simulink model "Simulation_Laboratory_Crazyflie2_X"  (R2015b)
settings: Solver=FixedStepAuto  SolverMode=SingleTasking  StartTime=0.0  StopTime=50  FixedStep=0.01  RelTol=1e-3
values from neighbouring files (symbols this model uses):
  fm = 0.2685    [CRAZYFLIE_SETUP.m]
  fs_inner = 50    [CRAZYFLIE_SETUP.m]
  fs_outer = 25    [CRAZYFLIE_SETUP.m]
  g = 9.81    [CRAZYFLIE_SETUP.m]
  Ixx = 1.657e-5    (= 1.657e-05)    [CRAZYFLIE_SETUP.m]
  Iyy = 1.665e-5    (= 1.665e-05)    [CRAZYFLIE_SETUP.m]
  Izz = 2.296e-5    (= 2.296e-05)    [CRAZYFLIE_SETUP.m]
  KDp = 2.5    [CRAZYFLIE_SETUP.m]
  KDphi = 0.3    [CRAZYFLIE_SETUP.m]
  KDq = 2.5    [CRAZYFLIE_SETUP.m]
  KDr = 2.5    [CRAZYFLIE_SETUP.m]
  KDtheta = 0.3    [CRAZYFLIE_SETUP.m]
  KIp = 500    [CRAZYFLIE_SETUP.m]
  KIphi = 0.3    [CRAZYFLIE_SETUP.m]
  KIq = 500    [CRAZYFLIE_SETUP.m]
  KIr = 500    [CRAZYFLIE_SETUP.m]
  KItheta = 0.3    [CRAZYFLIE_SETUP.m]
  KPp = 250    [CRAZYFLIE_SETUP.m]
  KPphi = 1.0    (= 1)    [CRAZYFLIE_SETUP.m]
  KPq = 250    [CRAZYFLIE_SETUP.m]
  KPr = 250    [CRAZYFLIE_SETUP.m]
  KPtheta = 1.0    (= 1)    [CRAZYFLIE_SETUP.m]
  m = 0.027    [CRAZYFLIE_SETUP.m]
  MCO1 = [1,-1/2,-1/2,-1 ... (first row only)    [CRAZYFLIE_SETUP.m]
  ML1 = 2*we*[CT,CT,CT,CT ... (first row only)    [CRAZYFLIE_SETUP.m]
  ML2 = [0,0 ... (first row only)    [CRAZYFLIE_SETUP.m]
  ML3 = [1/m;0]    [CRAZYFLIE_SETUP.m]
  ML4 = [0,0 ... (first row only)    [CRAZYFLIE_SETUP.m]
  ML5 = [1/Izz;0]    [CRAZYFLIE_SETUP.m]
  ML6 = [0,0,0,0 ... (first row only)    [CRAZYFLIE_SETUP.m]
  ML7 = [1/Ixx;0;0;0]    [CRAZYFLIE_SETUP.m]
  ML8 = [0,0,0,0 ... (first row only)    [CRAZYFLIE_SETUP.m]
  ML9 = [1/Iyy;0;0;0]    [CRAZYFLIE_SETUP.m]
  MNL1 = [CT,CT,CT,CT ... (first row only)    [CRAZYFLIE_SETUP.m]
  PWMe = (we-4070.3)/0.2685    [CRAZYFLIE_SETUP.m]
libraries: simulink x2
settings Model: Creator=Rafael  LastModifiedBy=Rafael
settings DataIOCC: SaveFormat=Array  SignalLoggingSaveFormat=ModelDataLogs
settings OptimizationCC: ExpressionDepthLimit=2147483647
settings DebuggingCC: UnderspecifiedInitializationDetection=Classic  MergeDetectMultiDrivingBlocksExec=none  SolverPrmCheckMsg=warning  FcnCallInpInsideContextMsg=EnableAllAsWarning  StateNameClashWarn=warning
settings HardwareCC: ProdBitPerPointer=32  ProdLargestAtomicFloat=None  ProdIntDivRoundTo=Undefined  ProdEndianess=Unspecified  ProdWordSize=32  ProdHWDeviceType=32-bit Generic
settings GRTTargetCC: GeneratePreprocessorConditionals=Disable all
settings ConfigComp: CovModelRefEnable=Off

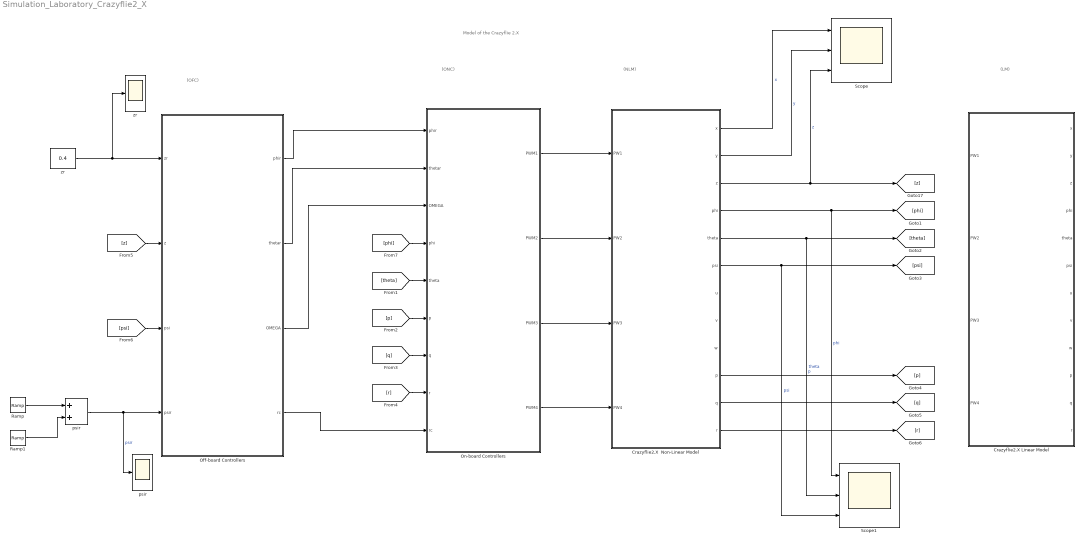
== system Simulation_Laboratory_Crazyflie2_X ==
  note: (NLM)
  note: Model of the Crazyflie 2.X
  note: (ONC)
  note: (LM)
  note: (OFC)
  " zr" : Scope
  Crazyflie2.X  Non-Linear Model : Subsystem
  Crazyflie2.X Linear Model : Subsystem
  Off-board Controllers : Subsystem
  On-board Controllers : Subsystem
  Ramp : simulink/Sources/Ramp  slope=15  start=5  X0=0
  Ramp1 : simulink/Sources/Ramp  slope=-15  start=11  X0=0
  Scope : Scope  NumInputPorts=3
  Scope1 : Scope  NumInputPorts=3
  psir : Sum
  "psir " : Scope
  zr : Constant  Value=0.4
  wires:
  [phi] -> On-board Controllers/4(phi)
  [theta] -> On-board Controllers/5(theta)
  [p] -> On-board Controllers/6(p)
  [q] -> On-board Controllers/7(q)
  [r] -> On-board Controllers/8(r)
  [z] -> Off-board Controllers/2(z)
  [psi] -> Off-board Controllers/3(psi)
  Crazyflie2.X  Non-Linear Model/11(q) -> [q]
  Crazyflie2.X  Non-Linear Model/3(z) -> [z], Scope/3  "z"
  Crazyflie2.X  Non-Linear Model/12(r) -> [r]
  zr/1 -> " zr"/1, Off-board Controllers/1(zr)
  Off-board Controllers/1(phir) -> On-board Controllers/1(phir)
  Crazyflie2.X  Non-Linear Model/10(p) -> [p]  "p"
  On-board Controllers/1(PWM1) -> Crazyflie2.X  Non-Linear Model/1(PW1)
  On-board Controllers/2(PWM2) -> Crazyflie2.X  Non-Linear Model/2(PW2)
  On-board Controllers/4(PWM4) -> Crazyflie2.X  Non-Linear Model/4(PW4)
  On-board Controllers/3(PWM3) -> Crazyflie2.X  Non-Linear Model/3(PW3)
  Crazyflie2.X  Non-Linear Model/4(phi) -> Scope1/1, [phi]  "phi"
  Crazyflie2.X  Non-Linear Model/5(theta) -> [theta], Scope1/2  "theta"
  Crazyflie2.X  Non-Linear Model/6(psi) -> [psi], Scope1/3  "psi"
  Off-board Controllers/2(thetar) -> On-board Controllers/2(thetar)
  Off-board Controllers/3(OMEGA) -> On-board Controllers/3(OMEGA)
  Off-board Controllers/4(rc) -> On-board Controllers/9(rc)
  Ramp/1 -> psir/1
  Ramp1/1 -> psir/2
  psir/1 -> "psir "/1, Off-board Controllers/4(psir)  "psir"
  Crazyflie2.X  Non-Linear Model/1(x) -> Scope/1  "x"
  Crazyflie2.X  Non-Linear Model/2(y) -> Scope/2  "y"

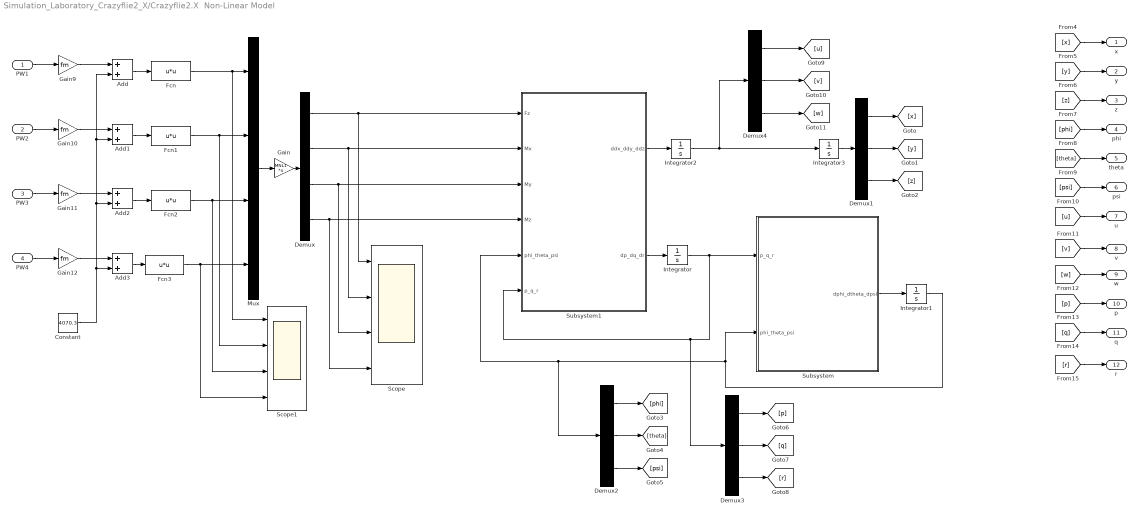
== system Simulation_Laboratory_Crazyflie2_X/Crazyflie2.X  Non-Linear Model ==
  PW1 : Inport
  PW2 : Inport  Port=2
  PW3 : Inport  Port=3
  PW4 : Inport  Port=4
  Add{,1..3} (4 alike) : Sum
  Constant : Constant  Value=4070.3
  Demux : Demux
  Demux{1..4} (4 alike) : Demux  Outputs=3
  Fcn{,1..3} (4 alike) : Fcn  Expr=u*u
  Gain : Gain  Gain=MNL1  Multiplication=Matrix(K*u) (u vector)
  Gain{9..12} (4 alike) : Gain  Gain=fm
  Integrator{,1..3} (4 alike) : Integrator
  Mux : Mux
  Scope : Scope  NumInputPorts=4
  Scope1 : Scope  NumInputPorts=4
  Subsystem : Subsystem
  Subsystem1 : Subsystem
  x : Outport
  y : Outport  Port=2
  z : Outport  Port=3
  phi : Outport  Port=4
  theta : Outport  Port=5
  psi : Outport  Port=6
  u : Outport  Port=7
  v : Outport  Port=8
  w : Outport  Port=9
  p : Outport  Port=10
  q : Outport  Port=11
  r : Outport  Port=12
  wires:
  Mux/1 -> Gain/1
  Gain/1 -> Demux/1
  Demux/1 -> Scope/1, Subsystem1/1(Fz)
  Demux/2 -> Scope/2, Subsystem1/2(Mx)
  Demux/3 -> Scope/3, Subsystem1/3(My)
  Demux/4 -> Scope/4, Subsystem1/4(Mz)
  [x] -> x/1
  [y] -> y/1
  [z] -> z/1
  [phi] -> phi/1
  [theta] -> theta/1
  [psi] -> psi/1
  [u] -> u/1
  [v] -> v/1
  [w] -> w/1
  [p] -> p/1
  [q] -> q/1
  [r] -> r/1
  PW1/1 -> Gain9/1
  PW2/1 -> Gain10/1
  PW3/1 -> Gain11/1
  PW4/1 -> Gain12/1
  Subsystem1/2(dp_dq_dr) -> Integrator/1
  Integrator/1 -> Subsystem/1(p_q_r), Subsystem1/6(p_q_r), Demux3/1
  Subsystem/1(dphi_dtheta_dpsi) -> Integrator1/1
  Integrator1/1 -> Subsystem/2(phi_theta_psi), Subsystem1/5(phi_theta_psi), Demux2/1
  Subsystem1/1(ddx_ddy_ddz) -> Integrator2/1
  Integrator2/1 -> Integrator3/1, Demux4/1
  Integrator3/1 -> Demux1/1
  Demux1/1 -> [x]
  Demux1/2 -> [y]
  Demux1/3 -> [z]
  Fcn/1 -> Mux/1, Scope1/1
  Fcn1/1 -> Mux/2, Scope1/2
  Fcn2/1 -> Mux/3, Scope1/3
  Fcn3/1 -> Mux/4, Scope1/4
  Demux2/1 -> [phi]
  Demux2/2 -> [theta]
  Demux2/3 -> [psi]
  Demux3/1 -> [p]
  Demux3/2 -> [q]
  Demux3/3 -> [r]
  Demux4/1 -> [u]
  Demux4/2 -> [v]
  Demux4/3 -> [w]
  Add/1 -> Fcn/1
  Add1/1 -> Fcn1/1
  Add2/1 -> Fcn2/1
  Add3/1 -> Fcn3/1
  Gain9/1 -> Add/1
  Gain10/1 -> Add1/1
  Gain11/1 -> Add2/1
  Gain12/1 -> Add3/1
  Constant/1 -> Add3/2, Add/2, Add1/2, Add2/2

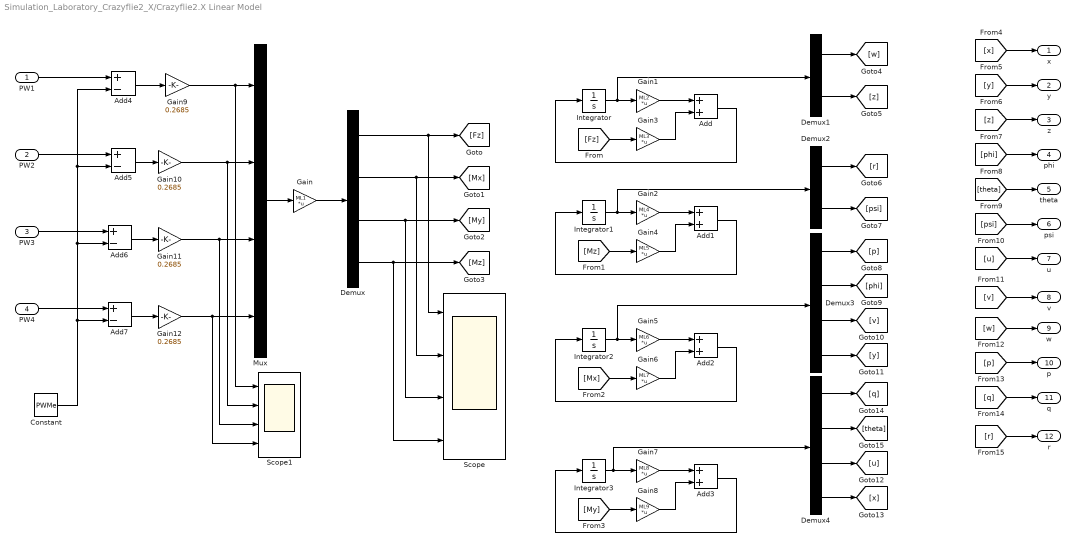
== system Simulation_Laboratory_Crazyflie2_X/Crazyflie2.X Linear Model ==
  PW1 : Inport
  PW2 : Inport  Port=2
  PW3 : Inport  Port=3
  PW4 : Inport  Port=4
  Add{,1..3} (4 alike) : Sum
  Add{4..7} (4 alike) : Sum  Inputs=+-
  Constant : Constant  Value=PWMe
  Demux : Demux
  Demux1 : Demux  Outputs=2
  Demux2 : Demux  Outputs=2
  Demux3 : Demux
  Demux4 : Demux
  Gain : Gain  Gain=ML1  Multiplication=Matrix(K*u) (u vector)
  Gain1 : Gain  Gain=ML2  Multiplication=Matrix(K*u) (u vector)
  Gain{9..12} (4 alike) : Gain  Gain=0.2685
  Gain2 : Gain  Gain=ML4  Multiplication=Matrix(K*u) (u vector)
  Gain3 : Gain  Gain=ML3  Multiplication=Matrix(K*u) (u vector)
  Gain4 : Gain  Gain=ML5  Multiplication=Matrix(K*u) (u vector)
  Gain5 : Gain  Gain=ML6  Multiplication=Matrix(K*u) (u vector)
  Gain6 : Gain  Gain=ML7  Multiplication=Matrix(K*u) (u vector)
  Gain7 : Gain  Gain=ML8  Multiplication=Matrix(K*u) (u vector)
  Gain8 : Gain  Gain=ML9  Multiplication=Matrix(K*u) (u vector)
  Integrator{,1..3} (4 alike) : Integrator
  Mux : Mux
  Scope : Scope  NumInputPorts=4
  Scope1 : Scope  NumInputPorts=4
  x : Outport
  y : Outport  Port=2
  z : Outport  Port=3
  phi : Outport  Port=4
  theta : Outport  Port=5
  psi : Outport  Port=6
  u : Outport  Port=7
  v : Outport  Port=8
  w : Outport  Port=9
  p : Outport  Port=10
  q : Outport  Port=11
  r : Outport  Port=12
  wires:
  Mux/1 -> Gain/1
  Gain/1 -> Demux/1
  Demux/1 -> [Fz], Scope/1
  Demux/2 -> [Mx], Scope/2
  Demux/3 -> [My], Scope/3
  Demux/4 -> [Mz], Scope/4
  Integrator/1 -> Gain1/1, Demux1/1
  [Fz] -> Gain3/1
  Gain1/1 -> Add/1
  Gain3/1 -> Add/2
  Add/1 -> Integrator/1
  Integrator1/1 -> Gain2/1, Demux2/1
  [Mz] -> Gain4/1
  Gain2/1 -> Add1/1
  Gain4/1 -> Add1/2
  Add1/1 -> Integrator1/1
  Integrator2/1 -> Gain5/1, Demux3/1
  [Mx] -> Gain6/1
  Gain5/1 -> Add2/1
  Gain6/1 -> Add2/2
  Add2/1 -> Integrator2/1
  Integrator3/1 -> Gain7/1, Demux4/1
  [My] -> Gain8/1
  Gain7/1 -> Add3/1
  Gain8/1 -> Add3/2
  Add3/1 -> Integrator3/1
  Demux1/1 -> [w]
  Demux1/2 -> [z]
  Demux2/2 -> [psi]
  Demux2/1 -> [r]
  Demux3/1 -> [p]
  Demux3/2 -> [phi]
  Demux3/3 -> [v]
  Demux3/4 -> [y]
  Demux4/1 -> [q]
  Demux4/2 -> [theta]
  Demux4/3 -> [u]
  Demux4/4 -> [x]
  [x] -> x/1
  [y] -> y/1
  [z] -> z/1
  [phi] -> phi/1
  [theta] -> theta/1
  [psi] -> psi/1
  [u] -> u/1
  [v] -> v/1
  [w] -> w/1
  [p] -> p/1
  [q] -> q/1
  [r] -> r/1
  PW1/1 -> Add4/1
  PW2/1 -> Add5/1
  PW3/1 -> Add6/1
  PW4/1 -> Add7/1
  Constant/1 -> Add4/2, Add5/2, Add6/2, Add7/2
  Add4/1 -> Gain9/1
  Gain9/1 -> Mux/1, Scope1/1
  Add5/1 -> Gain10/1
  Gain10/1 -> Mux/2, Scope1/2
  Add6/1 -> Gain11/1
  Gain11/1 -> Mux/3, Scope1/3
  Add7/1 -> Gain12/1
  Gain12/1 -> Mux/4, Scope1/4

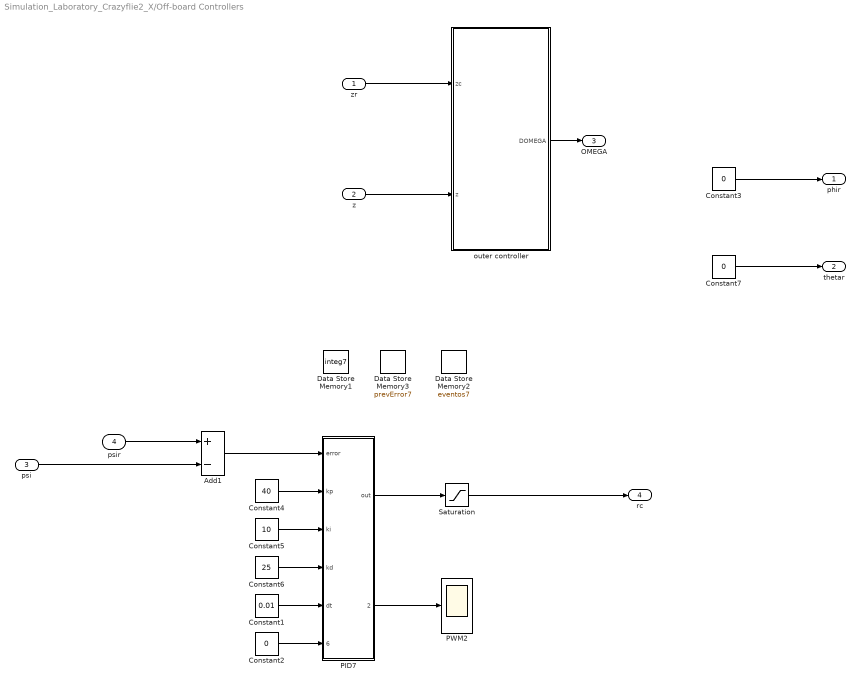
== system Simulation_Laboratory_Crazyflie2_X/Off-board Controllers ==
  zr : Inport
  z : Inport  Port=2
  psi : Inport  Port=3
  psir : Inport  Port=4
  Add1 : Sum  Inputs=+-
  Constant1 : Constant  Value=0.01
  Constant2 : Constant  Value=0
  Constant3 : Constant  Value=0
  Constant4 : Constant  Value=40
  Constant5 : Constant  Value=10
  Constant6 : Constant  Value=25
  Constant7 : Constant  Value=0
  Data Store Memory1 : DataStoreMemory  DataStoreName=integ7  ReadBeforeWriteMsg=warning  WriteAfterWriteMsg=warning  WriteAfterReadMsg=warning  OutDataTypeStr=double
  Data Store Memory2 : DataStoreMemory  DataStoreName=eventos7  ReadBeforeWriteMsg=warning  WriteAfterWriteMsg=warning  WriteAfterReadMsg=warning  OutDataTypeStr=double
  Data Store Memory3 : DataStoreMemory  DataStoreName=prevError7  ReadBeforeWriteMsg=warning  WriteAfterWriteMsg=warning  WriteAfterReadMsg=warning  OutDataTypeStr=double
  PID7 : MATLAB Function  TreatAsAtomicUnit=on
  PWM2 : Scope
  Saturation : Saturate  UpperLimit=20000  LowerLimit=-20000
  outer controller : Subsystem
  phir : Outport
  thetar : Outport  Port=2
  OMEGA : Outport  Port=3
  rc : Outport  Port=4
  wires:
  zr/1 -> outer controller/1(zc)
  z/1 -> outer controller/2(z)
  psi/1 -> Add1/2
  psir/1 -> Add1/1
  Constant1/1 -> PID7/5(dt)
  Constant6/1 -> PID7/4(kd)
  Constant4/1 -> PID7/2(kp)
  Constant5/1 -> PID7/3(ki)
  Add1/1 -> PID7/1(error)
  PID7/2(eventos) -> PWM2/1
  Constant2/1 -> PID7/6(umbral)
  PID7/1(out) -> Saturation/1
  Saturation/1 -> rc/1
  outer controller/1(DOMEGA) -> OMEGA/1
  Constant3/1 -> phir/1
  Constant7/1 -> thetar/1

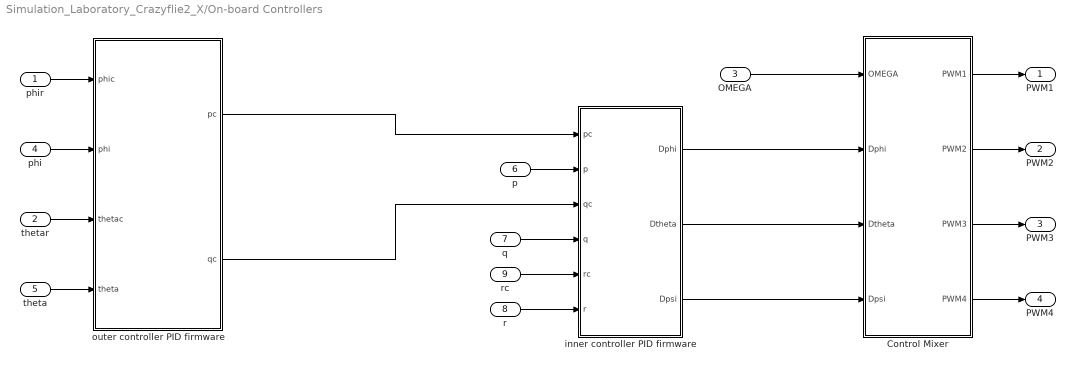
== system Simulation_Laboratory_Crazyflie2_X/On-board Controllers ==
  phir : Inport
  thetar : Inport  Port=2
  OMEGA : Inport  Port=3
  phi : Inport  Port=4
  theta : Inport  Port=5
  p : Inport  Port=6
  q : Inport  Port=7
  r : Inport  Port=8
  rc : Inport  Port=9
  Control Mixer : Subsystem
  inner controller PID firmware : Subsystem
  outer controller PID firmware : Subsystem
  PWM1 : Outport
  PWM2 : Outport  Port=2
  PWM3 : Outport  Port=3
  PWM4 : Outport  Port=4
  wires:
  phir/1 -> outer controller PID firmware/1(phic)
  thetar/1 -> outer controller PID firmware/3(thetac)
  phi/1 -> outer controller PID firmware/2(phi)
  theta/1 -> outer controller PID firmware/4(theta)
  Control Mixer/1(PWM1) -> PWM1/1
  Control Mixer/2(PWM2) -> PWM2/1
  Control Mixer/3(PWM3) -> PWM3/1
  Control Mixer/4(PWM4) -> PWM4/1
  OMEGA/1 -> Control Mixer/1(OMEGA)
  p/1 -> inner controller PID firmware/2(p)
  inner controller PID firmware/1(Dphi) -> Control Mixer/2(Dphi)
  q/1 -> inner controller PID firmware/4(q)
  inner controller PID firmware/2(Dtheta) -> Control Mixer/3(Dtheta)
  r/1 -> inner controller PID firmware/6(r)
  inner controller PID firmware/3(Dpsi) -> Control Mixer/4(Dpsi)
  rc/1 -> inner controller PID firmware/5(rc)
  outer controller PID firmware/1(pc) -> inner controller PID firmware/1(pc)
  outer controller PID firmware/2(qc) -> inner controller PID firmware/3(qc)

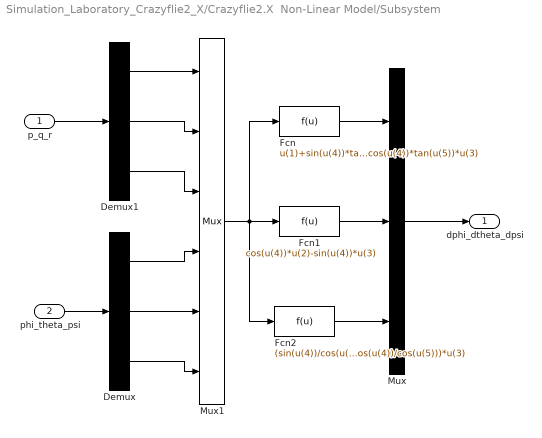
== system Simulation_Laboratory_Crazyflie2_X/Crazyflie2.X  Non-Linear Model/Subsystem ==
  p_q_r : Inport
  phi_theta_psi : Inport  Port=2
  Demux : Demux  Outputs=3
  Demux1 : Demux  Outputs=3
  Fcn : Fcn  Expr=u(1)+sin(u(4))*tan(u(5))*u(2)+cos(u(4))*tan(u(5))*u(3)
  Fcn1 : Fcn  Expr=cos(u(4))*u(2)-sin(u(4))*u(3)
  Fcn2 : Fcn  Expr=(sin(u(4))/cos(u(5)))*u(2)+(cos(u(4))/cos(u(5)))*u(3)
  Mux : Mux  Inputs=3
  Mux1 : Mux  Inputs=6
  dphi_dtheta_dpsi : Outport
  wires:
  Mux1/1 -> Fcn1/1, Fcn/1, Fcn2/1
  Fcn2/1 -> Mux/3
  Fcn/1 -> Mux/1
  Fcn1/1 -> Mux/2
  Mux/1 -> dphi_dtheta_dpsi/1
  Demux/3 -> Mux1/6
  Demux/2 -> Mux1/5
  Demux/1 -> Mux1/4
  Demux1/3 -> Mux1/3
  Demux1/2 -> Mux1/2
  Demux1/1 -> Mux1/1
  phi_theta_psi/1 -> Demux/1
  p_q_r/1 -> Demux1/1

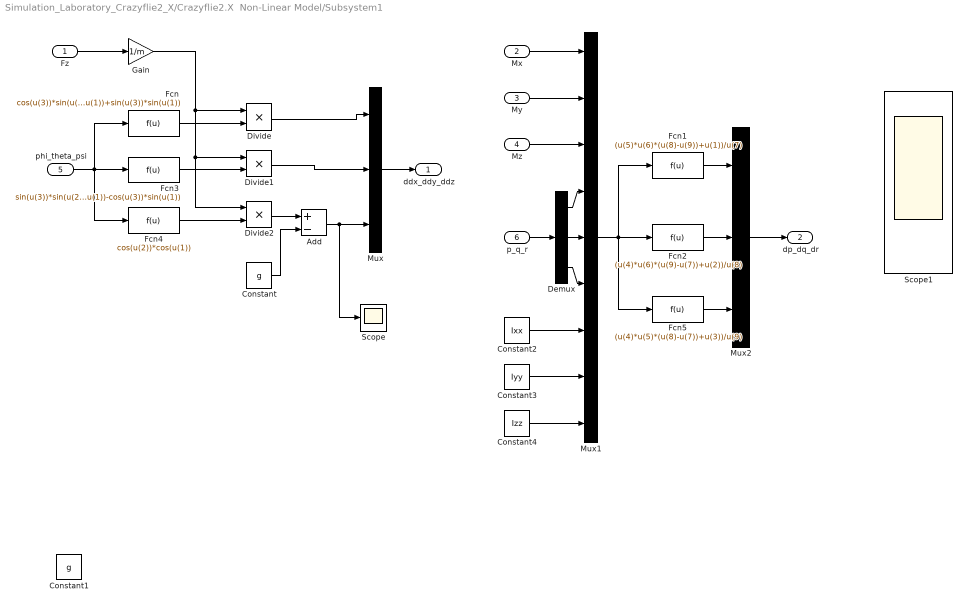
== system Simulation_Laboratory_Crazyflie2_X/Crazyflie2.X  Non-Linear Model/Subsystem1 ==
  Fz : Inport
  Mx : Inport  Port=2
  My : Inport  Port=3
  Mz : Inport  Port=4
  phi_theta_psi : Inport  Port=5
  p_q_r : Inport  Port=6
  Add : Sum  Inputs=+-
  Constant : Constant  Value=g
  Constant1 : Constant  Value=g
  Constant2 : Constant  Value=Ixx
  Constant3 : Constant  Value=Iyy
  Constant4 : Constant  Value=Izz
  Demux : Demux  Outputs=3
  Divide : Product  Inputs=**
  Divide1 : Product  Inputs=**
  Divide2 : Product  Inputs=**
  Fcn : Fcn  Expr=cos(u(3))*sin(u(2))*cos(u(1))+sin(u(3))*sin(u(1))
  Fcn1 : Fcn  Expr=(u(5)*u(6)*(u(8)-u(9))+u(1))/u(7)
  Fcn2 : Fcn  Expr=(u(4)*u(6)*(u(9)-u(7))+u(2))/u(8)
  Fcn3 : Fcn  Expr=sin(u(3))*sin(u(2))*sin(u(1))-cos(u(3))*sin(u(1))
  Fcn4 : Fcn  Expr=cos(u(2))*cos(u(1))
  Fcn5 : Fcn  Expr=(u(4)*u(5)*(u(8)-u(7))+u(3))/u(9)
  Gain : Gain  Gain=1/m
  Mux : Mux  Inputs=3
  Mux1 : Mux  Inputs=9
  Mux2 : Mux  Inputs=3
  Scope : Scope
  Scope1 : Scope  NumInputPorts=3
  ddx_ddy_ddz : Outport
  dp_dq_dr : Outport  Port=2
  wires:
  Mux/1 -> ddx_ddy_ddz/1
  Fz/1 -> Gain/1
  phi_theta_psi/1 -> Fcn/1, Fcn3/1, Fcn4/1
  Fcn/1 -> Divide/2
  Gain/1 -> Divide/1, Divide1/1, Divide2/1
  Fcn3/1 -> Divide1/2
  Fcn4/1 -> Divide2/2
  Divide2/1 -> Add/1
  Constant/1 -> Add/2
  Divide/1 -> Mux/1
  Divide1/1 -> Mux/2
  Add/1 -> Mux/3, Scope/1
  p_q_r/1 -> Demux/1
  Mx/1 -> Mux1/1
  My/1 -> Mux1/2
  Demux/2 -> Mux1/5
  Mz/1 -> Mux1/3
  Demux/1 -> Mux1/4
  Demux/3 -> Mux1/6
  Constant4/1 -> Mux1/9
  Constant3/1 -> Mux1/8
  Constant2/1 -> Mux1/7
  Mux2/1 -> dp_dq_dr/1
  Fcn1/1 -> Mux2/1
  Fcn2/1 -> Mux2/2
  Fcn5/1 -> Mux2/3
  Mux1/1 -> Fcn1/1, Fcn2/1, Fcn5/1

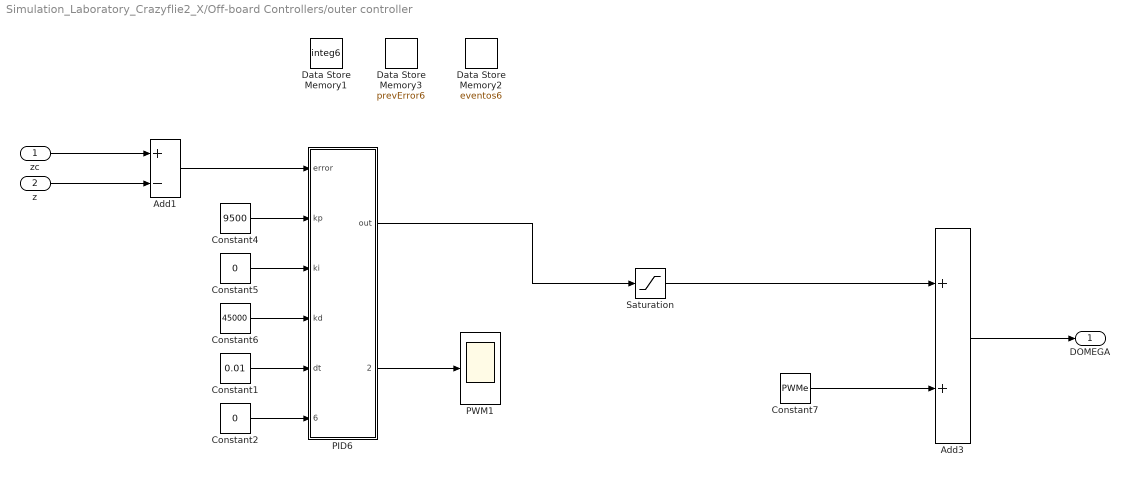
== system Simulation_Laboratory_Crazyflie2_X/Off-board Controllers/outer controller ==
  zc : Inport
  z : Inport  Port=2
  Add1 : Sum  Inputs=+-
  Add3 : Sum
  Constant1 : Constant  Value=0.01
  Constant2 : Constant  Value=0
  Constant4 : Constant  Value=9500
  Constant5 : Constant  Value=0
  Constant6 : Constant  Value=45000
  Constant7 : Constant  Value=PWMe
  Data Store Memory1 : DataStoreMemory  DataStoreName=integ6  ReadBeforeWriteMsg=warning  WriteAfterWriteMsg=warning  WriteAfterReadMsg=warning  OutDataTypeStr=double
  Data Store Memory2 : DataStoreMemory  DataStoreName=eventos6  ReadBeforeWriteMsg=warning  WriteAfterWriteMsg=warning  WriteAfterReadMsg=warning  OutDataTypeStr=double
  Data Store Memory3 : DataStoreMemory  DataStoreName=prevError6  ReadBeforeWriteMsg=warning  WriteAfterWriteMsg=warning  WriteAfterReadMsg=warning  OutDataTypeStr=double
  PID6 : MATLAB Function  TreatAsAtomicUnit=on
  PWM1 : Scope
  Saturation : Saturate  UpperLimit=20000  LowerLimit=-20000
  DOMEGA : Outport
  wires:
  Add3/1 -> DOMEGA/1
  Constant7/1 -> Add3/2
  zc/1 -> Add1/1
  z/1 -> Add1/2
  Constant1/1 -> PID6/5(dt)
  Constant6/1 -> PID6/4(kd)
  Constant4/1 -> PID6/2(kp)
  Constant5/1 -> PID6/3(ki)
  Add1/1 -> PID6/1(error)
  Saturation/1 -> Add3/1
  PID6/2(eventos) -> PWM1/1
  Constant2/1 -> PID6/6(umbral)
  PID6/1(out) -> Saturation/1

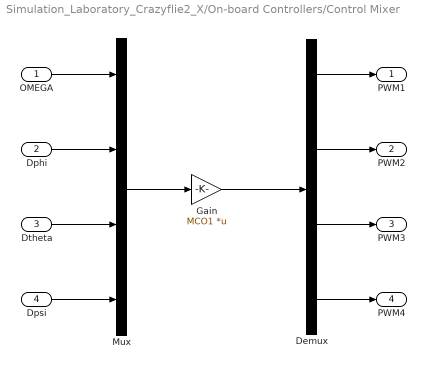
== system Simulation_Laboratory_Crazyflie2_X/On-board Controllers/Control Mixer ==
  OMEGA : Inport
  Dphi : Inport  Port=2
  Dtheta : Inport  Port=3
  Dpsi : Inport  Port=4
  Demux : Demux
  Gain : Gain  Gain=MCO1  Multiplication=Matrix(K*u) (u vector)
  Mux : Mux
  PWM1 : Outport
  PWM2 : Outport  Port=2
  PWM3 : Outport  Port=3
  PWM4 : Outport  Port=4
  wires:
  OMEGA/1 -> Mux/1
  Dphi/1 -> Mux/2
  Dtheta/1 -> Mux/3
  Dpsi/1 -> Mux/4
  Demux/4 -> PWM4/1
  Demux/3 -> PWM3/1
  Demux/2 -> PWM2/1
  Demux/1 -> PWM1/1
  Gain/1 -> Demux/1
  Mux/1 -> Gain/1

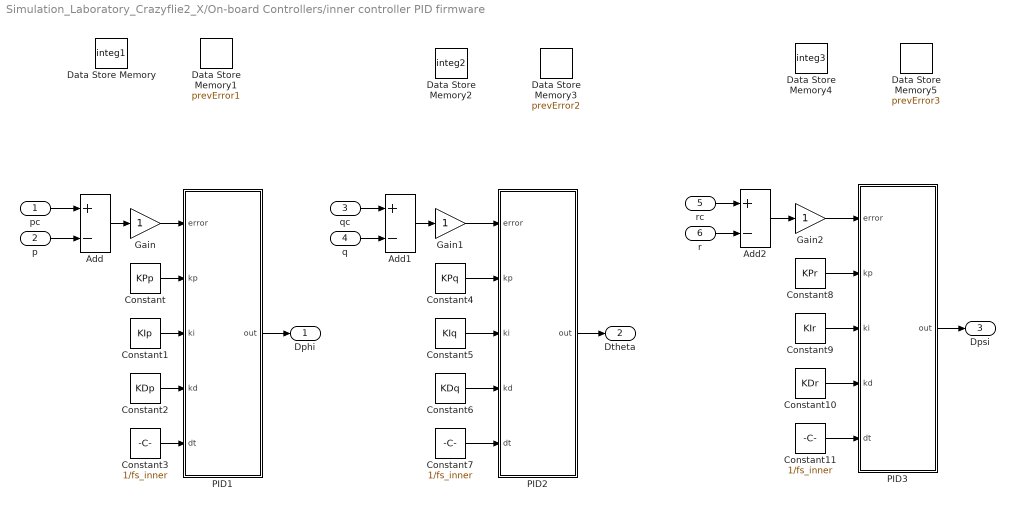
== system Simulation_Laboratory_Crazyflie2_X/On-board Controllers/inner controller PID firmware ==
  pc : Inport
  p : Inport  Port=2
  qc : Inport  Port=3
  q : Inport  Port=4
  rc : Inport  Port=5
  r : Inport  Port=6
  Add : Sum  Inputs=+-
  Add1 : Sum  Inputs=+-
  Add2 : Sum  Inputs=+-
  Constant : Constant  Value=KPp
  Constant1 : Constant  Value=KIp
  Constant10 : Constant  Value=KDr
  Constant11 : Constant  Value=1/fs_inner
  Constant2 : Constant  Value=KDp
  Constant3 : Constant  Value=1/fs_inner
  Constant4 : Constant  Value=KPq
  Constant5 : Constant  Value=KIq
  Constant6 : Constant  Value=KDq
  Constant7 : Constant  Value=1/fs_inner
  Constant8 : Constant  Value=KPr
  Constant9 : Constant  Value=KIr
  Data Store Memory : DataStoreMemory  DataStoreName=integ1  ReadBeforeWriteMsg=warning  WriteAfterWriteMsg=warning  WriteAfterReadMsg=warning  OutDataTypeStr=double
  Data Store Memory1 : DataStoreMemory  DataStoreName=prevError1  ReadBeforeWriteMsg=warning  WriteAfterWriteMsg=warning  WriteAfterReadMsg=warning  OutDataTypeStr=double
  Data Store Memory2 : DataStoreMemory  DataStoreName=integ2  ReadBeforeWriteMsg=warning  WriteAfterWriteMsg=warning  WriteAfterReadMsg=warning  OutDataTypeStr=double
  Data Store Memory3 : DataStoreMemory  DataStoreName=prevError2  ReadBeforeWriteMsg=warning  WriteAfterWriteMsg=warning  WriteAfterReadMsg=warning  OutDataTypeStr=double
  Data Store Memory4 : DataStoreMemory  DataStoreName=integ3  ReadBeforeWriteMsg=warning  WriteAfterWriteMsg=warning  WriteAfterReadMsg=warning  OutDataTypeStr=double
  Data Store Memory5 : DataStoreMemory  DataStoreName=prevError3  ReadBeforeWriteMsg=warning  WriteAfterWriteMsg=warning  WriteAfterReadMsg=warning  OutDataTypeStr=double
  Gain : Gain  SampleTime=1/fs_inner
  Gain1 : Gain  SampleTime=1/fs_inner
  Gain2 : Gain  SampleTime=1/fs_inner
  PID1 : MATLAB Function  TreatAsAtomicUnit=on
  PID2 : MATLAB Function  TreatAsAtomicUnit=on
  PID3 : MATLAB Function  TreatAsAtomicUnit=on
  Dphi : Outport
  Dtheta : Outport  Port=2
  Dpsi : Outport  Port=3
  wires:
  pc/1 -> Add/1
  p/1 -> Add/2
  qc/1 -> Add1/1
  q/1 -> Add1/2
  rc/1 -> Add2/1
  r/1 -> Add2/2
  Add/1 -> Gain/1
  Gain/1 -> PID1/1(error)
  PID1/1(out) -> Dphi/1
  Constant/1 -> PID1/2(kp)
  Constant1/1 -> PID1/3(ki)
  Constant2/1 -> PID1/4(kd)
  Add1/1 -> Gain1/1
  Constant3/1 -> PID1/5(dt)
  Gain1/1 -> PID2/1(error)
  PID2/1(out) -> Dtheta/1
  Constant4/1 -> PID2/2(kp)
  Constant5/1 -> PID2/3(ki)
  Constant6/1 -> PID2/4(kd)
  Constant7/1 -> PID2/5(dt)
  Gain2/1 -> PID3/1(error)
  PID3/1(out) -> Dpsi/1
  Constant8/1 -> PID3/2(kp)
  Constant9/1 -> PID3/3(ki)
  Constant10/1 -> PID3/4(kd)
  Constant11/1 -> PID3/5(dt)
  Add2/1 -> Gain2/1

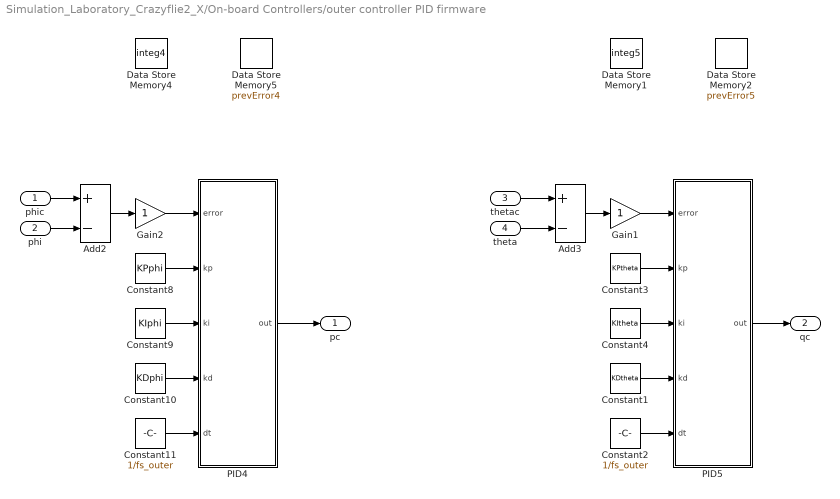
== system Simulation_Laboratory_Crazyflie2_X/On-board Controllers/outer controller PID firmware ==
  phic : Inport
  phi : Inport  Port=2
  thetac : Inport  Port=3
  theta : Inport  Port=4
  Add2 : Sum  Inputs=+-
  Add3 : Sum  Inputs=+-
  Constant1 : Constant  Value=KDtheta
  Constant10 : Constant  Value=KDphi
  Constant11 : Constant  Value=1/fs_outer
  Constant2 : Constant  Value=1/fs_outer
  Constant3 : Constant  Value=KPtheta
  Constant4 : Constant  Value=KItheta
  Constant8 : Constant  Value=KPphi
  Constant9 : Constant  Value=KIphi
  Data Store Memory1 : DataStoreMemory  DataStoreName=integ5  ReadBeforeWriteMsg=warning  WriteAfterWriteMsg=warning  WriteAfterReadMsg=warning  OutDataTypeStr=double
  Data Store Memory2 : DataStoreMemory  DataStoreName=prevError5  ReadBeforeWriteMsg=warning  WriteAfterWriteMsg=warning  WriteAfterReadMsg=warning  OutDataTypeStr=double
  Data Store Memory4 : DataStoreMemory  DataStoreName=integ4  ReadBeforeWriteMsg=warning  WriteAfterWriteMsg=warning  WriteAfterReadMsg=warning  OutDataTypeStr=double
  Data Store Memory5 : DataStoreMemory  DataStoreName=prevError4  ReadBeforeWriteMsg=warning  WriteAfterWriteMsg=warning  WriteAfterReadMsg=warning  OutDataTypeStr=double
  Gain1 : Gain  SampleTime=1/fs_outer
  Gain2 : Gain  SampleTime=1/fs_outer
  PID4 : MATLAB Function  TreatAsAtomicUnit=on
  PID5 : MATLAB Function  TreatAsAtomicUnit=on
  pc : Outport
  qc : Outport  Port=2
  wires:
  thetac/1 -> Add3/1
  theta/1 -> Add3/2
  Gain2/1 -> PID4/1(error)
  Constant8/1 -> PID4/2(kp)
  Constant9/1 -> PID4/3(ki)
  Constant10/1 -> PID4/4(kd)
  Constant11/1 -> PID4/5(dt)
  Add2/1 -> Gain2/1
  phic/1 -> Add2/1
  phi/1 -> Add2/2
  Gain1/1 -> PID5/1(error)
  Constant3/1 -> PID5/2(kp)
  Constant4/1 -> PID5/3(ki)
  Constant1/1 -> PID5/4(kd)
  Constant2/1 -> PID5/5(dt)
  Add3/1 -> Gain1/1
  PID5/1(out) -> qc/1
  PID4/1(out) -> pc/1

== matlab function Simulation_Laboratory_Crazyflie2_X/On-board Controllers/inner controller PID firmware/PID2 ==
  data: error input; out output; kp input; ki input; kd input; dt input; integ2 data_store_memory; prevError2 data_store_memory
function out = fcn(error,kp,ki,kd,dt)
%#codegen
global integ2;
global prevError2;
integ2=integ2+error*dt;
deriv=(error-prevError2)/dt;
outP=kp*error;
outI=ki*integ2;
outD=kd*deriv;
prevError2=error;
out = outP+outI+outD;

== matlab function Simulation_Laboratory_Crazyflie2_X/On-board Controllers/inner controller PID firmware/PID1 ==
  data: error input; out output; kp input; ki input; kd input; dt input; integ1 data_store_memory; prevError1 data_store_memory
function out = fcn(error,kp,ki,kd,dt)
%#codegen
global integ1;
global prevError1;
integ1=integ1+error*dt;
deriv=(error-prevError1)/dt;
outP=kp*error;
outI=ki*integ1;
outD=kd*deriv;
prevError1=error;
out = outP+outI+outD;

== matlab function Simulation_Laboratory_Crazyflie2_X/On-board Controllers/inner controller PID firmware/PID3 ==
  data: error input; out output; kp input; ki input; kd input; dt input; integ3 data_store_memory; prevError3 data_store_memory
function out = fcn(error,kp,ki,kd,dt)
%#codegen
global integ3;
global prevError3;
integ3=integ3+error*dt;
deriv=(error-prevError3)/dt;
outP=kp*error;
outI=ki*integ3;
outD=kd*deriv;
prevError3=error;
out = outP+outI+outD;

== matlab function Simulation_Laboratory_Crazyflie2_X/On-board Controllers/outer controller PID firmware/PID4 ==
  data: error input; out output; kp input; ki input; kd input; dt input; integ4 data_store_memory; prevError4 data_store_memory
function out = fcn(error,kp,ki,kd,dt)
%#codegen
global integ4;
global prevError4;
integ4=integ4+error*dt;
deriv=(error-prevError4)/dt;
outP=kp*error;
outI=ki*integ4;
outD=kd*deriv;
prevError4=error;
out = outP+outI+outD;

== matlab function Simulation_Laboratory_Crazyflie2_X/On-board Controllers/outer controller PID firmware/PID5 ==
  data: error input; out output; kp input; ki input; kd input; dt input; integ5 data_store_memory; prevError5 data_store_memory
function out = fcn(error,kp,ki,kd,dt)
%#codegen
global integ5;
global prevError5;
integ5=integ5+error*dt;
deriv=(error-prevError5)/dt;
outP=kp*error;
outI=ki*integ5;
outD=kd*deriv;
prevError5=error;
out = outP+outI+outD;

== matlab function Simulation_Laboratory_Crazyflie2_X/Off-board Controllers/PID7 ==
  data: out output; error input; kp input; ki input; kd input; dt input; eventos output; umbral input; integ7 data_store_memory; prevError7 data_store_memory; eventos7 data_store_memory
function [out,eventos] = fcn(error,kp,ki,kd,dt,umbral)
%#codegen
global integ7;
global prevError7;
global eventos7;
integ7=integ7+error*dt;
deriv=(error-prevError7)/dt;
outP=0;
outI=ki*integ7;
outD=kd*deriv;
prevError7=error;
if (abs(error)>umbral)
    eventos7=eventos7+1;
    outP=kp*error;
end
out = outP+outI+outD;
eventos=eventos7;

== matlab function Simulation_Laboratory_Crazyflie2_X/Off-board Controllers/outer controller/PID6 ==
  data: out output; error input; kp input; ki input; kd input; dt input; integ6 data_store_memory; prevError6 data_store_memory; eventos output; umbral input; eventos6 data_store_memory
function [out,eventos] = fcn(error,kp,ki,kd,dt,umbral)
%#codegen
global integ6;
global prevError6;
global eventos6;
integ6=integ6+error*dt;
deriv=(error-prevError6)/dt;
outP=kp*error;
outI=ki*integ6;
outD=0;
prevError6=error;
if (abs(error)>umbral)
    eventos6=eventos6+1;
    outD=kd*deriv;
end
out = outP+outI+outD;
eventos=eventos6;
